simulink library "wingController"  (R2018a)
settings: Solver=VariableStepAuto  StartTime=0.0  StopTime=10.0  RelTol=1e-3
undefined symbols (not defined in the file): iterationPhase_enum
libraries: calculateFeatheredWingAngle x1, calculateOptimalWingAngle x1, simulink x1, saturateWingAngle x1
settings Model: Creator=mitch  LastModifiedBy=mitch

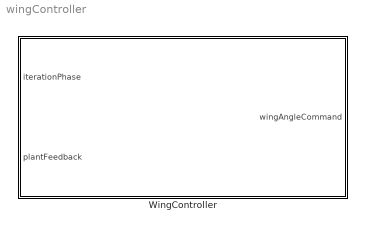
== system wingController ==
  WingController : Subsystem

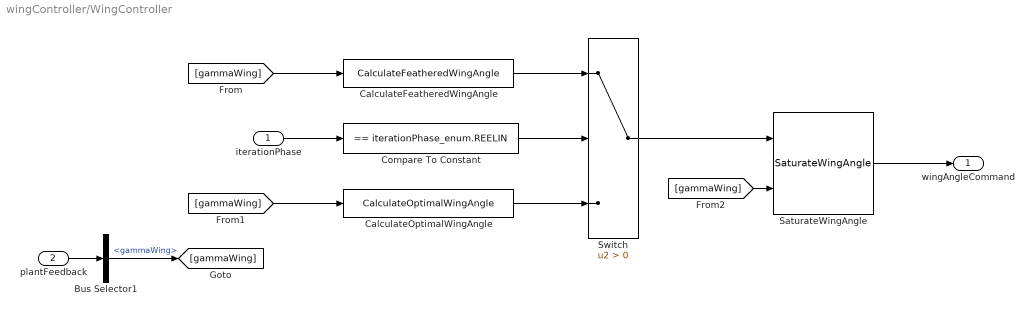
== system wingController/WingController ==
  iterationPhase : Inport
  plantFeedback : Inport  Port=2
  Bus Selector1 : BusSelector  OutputSignals=gammaWing
  CalculateFeatheredWingAngle : calculateFeatheredWingAngle/CalculateFeatheredWingAngle
  CalculateOptimalWingAngle : calculateOptimalWingAngle/CalculateOptimalWingAngle
  Compare To Constant : simulink/Logic and Bit Operations/Compare To Constant  relop===  const=iterationPhase_enum.REELIN  OutDataTypeStr=boolean
  SaturateWingAngle : saturateWingAngle/SaturateWingAngle
  Switch : Switch  Criteria=u2 > Threshold
  wingAngleCommand : Outport
  wires:
  plantFeedback/1 -> Bus Selector1/1
  SaturateWingAngle/1 -> wingAngleCommand/1
  iterationPhase/1 -> Compare To Constant/1
  Compare To Constant/1 -> Switch/2
  CalculateFeatheredWingAngle/1 -> Switch/1
  CalculateOptimalWingAngle/1 -> Switch/3
  Switch/1 -> SaturateWingAngle/1
  Bus Selector1/1 -> [gammaWing]  "<gammaWing>"
  [gammaWing] -> CalculateFeatheredWingAngle/1
  [gammaWing] -> CalculateOptimalWingAngle/1
  [gammaWing] -> SaturateWingAngle/2
